simulink library "Slope_Resistance"  (R2018b)
settings: Solver=VariableStepAuto  StartTime=0.0  StopTime=10.0  RelTol=1e-3
settings Model: Creator=Alexander Koch  LastModifiedBy=ga69qig
settings SFSimCC: SimUseLocalCustomCode=off
settings RTWCC: RTWUseLocalCustomCode=off
settings CodeAppCC: StateflowObjectComments=on

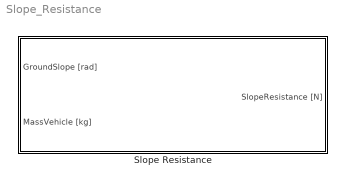
== system Slope_Resistance ==
  Slope Resistance : Subsystem  mask(SB){Gravity=9.81, LocalSampleTime=-1}
      mask prompts: Gravity "Gravity [N/kg]"; LocalSampleTime "Local System Sample-Time [s]"
      mask help:
      | <Author> Alexander Koch, Benedikt Danquah based on Stefan Müller [1], Stephan Rohr [2]  </Author>
      | <Date> 21/03/2017 </Date>
      | <Sources>
      | [1] S. Mueller, S. Rohr, und et al, Hrsg, Analysing the Influence of Driver Behaviour and Tuning Measures on Battery Aging and Residual Value of Electric Vehicles, 2017
      | </Sources>
      |
      | <Description>
      | Requires ground slope, mass of the vehicle and gravity and calculates the slope resistance.
      | </Description>
      mask init:
      | GlobalSampleTime = CalcGlobalSampleTime(LocalSampleTime);
      mask Help:
      | <Parameters>
      | Gravity [N/kg]
      | Local System Sample-Time [s]
      | 	<Min> GlobalSampleTime </Min>
      | Global Sample-Time [s]
      | </Parameters>
      | 
      | <Inputs>
      | GroundSlope [rad]
      | 	<sign orientation> [+] uphill </sign orientation>
      | MassVehicle [kg]
      | </Inputs>
      | 
      | <Outputs>
      | SlopeResistance [N]
      | </Outputs>
      | <Sources>
      | [1] S. Mueller, S. Rohr, W. Schmid, and M. Lienkamp, “Analysing the Influence of Driver Behaviour and Tuning Measures on Battery Aging and Residual Value of Electric Vehicles,” in Proc. EVS30 Symposium, Stuttgart, 2017, pp. 1–12.
      | [2] S. Rohr, “Technisch-wirtschaftliche Analyse des Zweitnutzungs- potentials von Lithium-Ionen-Traktionsbatterien,” Dissertation, Institute of Automotive Technology, Technical University Munich, Munich, 2018.
      | </Sources>
      mask TypeOptions Gravity: Gravity/Gain
      mask TypeOptions LocalSampleTime: GroundSlope [rad]/SampleTime | MassVehicle [kg]/SampleTime
      mask DialogControl Container3 Prompt: Documentation:
      mask DialogControl Control2 Prompt: %<MaskHelp>
      mask DialogControl Container5 Prompt: Sample Time
      mask Display:
      | [picturexpos,pictureypos,picturewidth,pictureheight] = ...
      |     CalcBlockPicturePosition(gcb,8.5/6.5,0.01,0.1,90,90); % calculating picture position depending on Block size and minimum margin size
      | image('Slope_Resistance.svg',[picturexpos pictureypos picturewidth pictureheight]); % plot picture to block

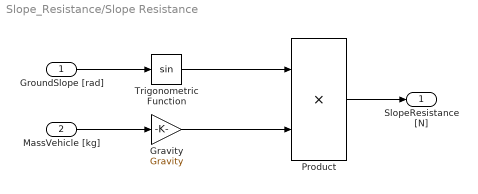
== system Slope_Resistance/Slope Resistance ==
  GroundSlope [rad] : Inport  SampleTime=LocalSampleTime
  MassVehicle [kg] : Inport  Port=2  SampleTime=LocalSampleTime
  Gravity : Gain  Gain=Gravity
  Product : Product
  Trigonometric Function : Trigonometry
  SlopeResistance [N] : Outport  SampleTime=GlobalSampleTime
  wires:
  Trigonometric Function/1 -> Product/1
  Gravity/1 -> Product/2
  MassVehicle [kg]/1 -> Gravity/1
  GroundSlope [rad]/1 -> Trigonometric Function/1
  Product/1 -> SlopeResistance [N]/1
